simulink model "imc_Q_d"  (Simulink 5.0)
settings: Solver=ode45  StartTime=t0  StopTime=tf  RelTol=1e-3
values from neighbouring files (symbols this model uses):
  alpha = 0.5    [lewin_imc.m]    (also in vande_imc1.m = 0.9)
  Ap = A    [lewin_imc.m]    (also in vande_imc1.m)
  Bp = B    [lewin_imc.m]    (also in vande_imc1.m)
  Nvar = 0    [vande_imc1.m]
  st = 1    [vande_imc1.m]
  Ts = 3    [lewin_imc.m]    (also in vande_imc1.m = 0.1)
undefined symbols (not defined in the file or in its folder): A, B, GiD, GiN, zk
settings Model: Creator=kannanm  LastModifiedBy=kannan  ExtModeAutoUpdateStatusClock=off

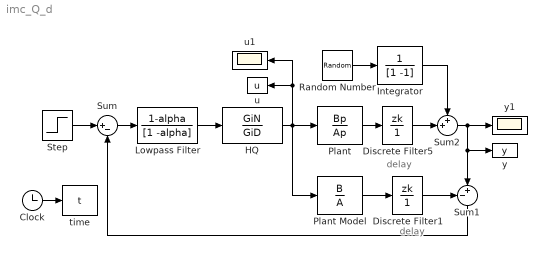
== system imc_Q_d ==
  note: delay
  note: delay
  Clock : Clock
      settings: Decimation=10
  Discrete Filter1 : DiscreteFilter  Numerator=zk  Denominator=1  SampleTime=Ts
  Discrete Filter5 : DiscreteFilter  Numerator=zk  Denominator=1  SampleTime=Ts
  HQ : DiscreteFilter  Numerator=GiN  Denominator=GiD  SampleTime=Ts
  Integrator : DiscreteFilter  Numerator=1  Denominator=[1 -1]  SampleTime=Ts
  Lowpass Filter : DiscreteFilter  Numerator=1-alpha  Denominator=[1 -alpha]  SampleTime=Ts
  Plant : DiscreteFilter  Numerator=Bp  Denominator=Ap  SampleTime=Ts
  Plant Model : DiscreteFilter  Numerator=B  Denominator=A  SampleTime=Ts
  Random Number : RandomNumber  Variance=Nvar  SampleTime=Ts
  Step : Step  After=st  SampleTime=Ts
  Sum : Sum  Inputs=|+-  SaturateOnIntegerOverflow=on
  Sum1 : Sum  Orientation=down  Inputs=-+|  SaturateOnIntegerOverflow=on
  Sum2 : Sum  Inputs=++|  SaturateOnIntegerOverflow=on
  time : ToWorkspace  VariableName=t  SampleTime=Ts  SaveFormat=Array
  u : ToWorkspace  VariableName=u  SampleTime=Ts  SaveFormat=Array
  u1 : Scope
  y : ToWorkspace  VariableName=y  SampleTime=Ts  SaveFormat=Array
  y1 : Scope
  wires:
  Lowpass Filter/1 -> HQ/1
  HQ/1 -> Plant/1, Plant Model/1, u1/1, u/1
  Sum/1 -> Lowpass Filter/1
  Plant Model/1 -> Discrete Filter1/1
  Plant/1 -> Discrete Filter5/1
  Sum1/1 -> Sum/2
  Step/1 -> Sum/1
  Integrator/1 -> Sum2/1
  Sum2/1 -> y1/1, Sum1/2, y/1
  Discrete Filter5/1 -> Sum2/2
  Discrete Filter1/1 -> Sum1/1
  Random Number/1 -> Integrator/1
  Clock/1 -> time/1
